simulink subsystem "Cell"  (R2019b)
settings: Solver=VariableStepAuto  StartTime=0.0  StopTime=10.0  RelTol=1e-3
libraries: nesl_utility x12, fl_lib x11, ee_lib x2
settings Model: Creator=PcElettronicaDynamis  LastModifiedBy=PcElettronicaDynamis

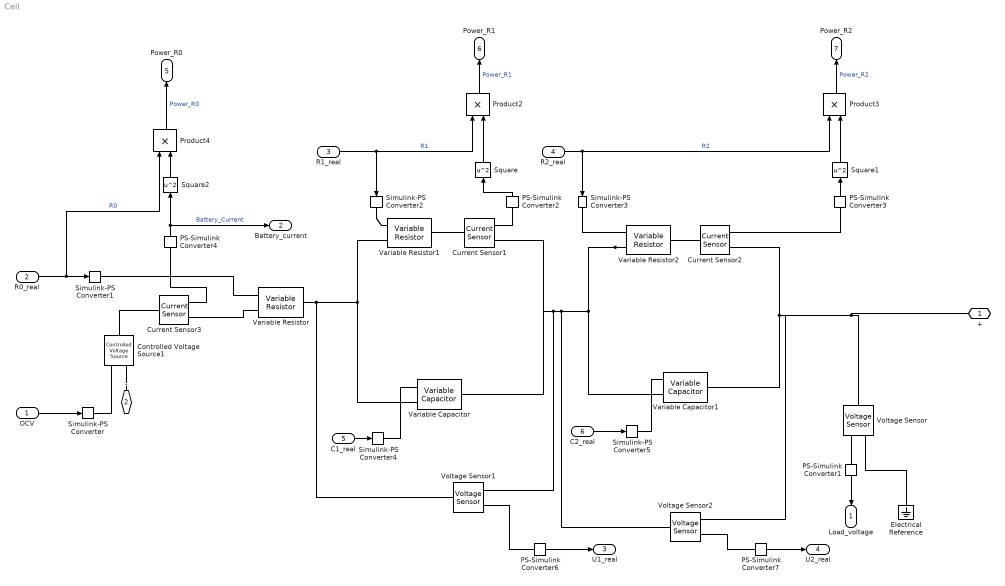
== system Cell ==
  OCV : Inport
  R0_real : Inport  Port=2
  R1_real : Inport  Port=3
  R2_real : Inport  Port=4
  C1_real : Inport  Port=5
  C2_real : Inport  Port=6
  Controlled Voltage Source1 : fl_lib/Electrical/Electrical Sources/Controlled Voltage Source
  Current Sensor1 : fl_lib/Electrical/Electrical Sensors/Current Sensor
  Current Sensor2 : fl_lib/Electrical/Electrical Sensors/Current Sensor
  Current Sensor3 : fl_lib/Electrical/Electrical Sensors/Current Sensor
  Electrical Reference : fl_lib/Electrical/Electrical Elements/Electrical Reference
  PS-Simulink Converter{1..4} (4 alike) : nesl_utility/PS-Simulink Converter  PhysicalDomain=network_engine_domain  SubClassName=ps_output  LeftPortType=input  RightPortType=output  PseudoPeriodic=off  Frequencies=[]  Unit=1  AffineConversion=off
  PS-Simulink Converter6 : nesl_utility/PS-Simulink Converter  PhysicalDomain=network_engine_domain  SubClassName=ps_output  LeftPortType=input  RightPortType=output  PseudoPeriodic=off  Frequencies=[]  Unit=inherit  AffineConversion=off
  PS-Simulink Converter7 : nesl_utility/PS-Simulink Converter  PhysicalDomain=network_engine_domain  SubClassName=ps_output  LeftPortType=input  RightPortType=output  PseudoPeriodic=off  Frequencies=[]  Unit=inherit  AffineConversion=off
  Product2 : Product
  Product3 : Product
  Product4 : Product
  Simulink-PS Converter{,1..5} (6 alike) : nesl_utility/Simulink-PS Converter  PhysicalDomain=network_engine_domain  SubClassName=ps_input  LeftPortType=input  RightPortType=output  PseudoPeriodic=off  Frequencies=[]  NoiseDistribution=none  NoiseParameters=[]  Unit=1  AffineConversion=off  FilteringAndDerivatives=provide  SimscapeFilterOrder=1  InputFilterTimeConstant=0.001  UdotUserProvided=0
  Square : Math  Operator=square  SaturateOnIntegerOverflow=on
  Square1 : Math  Operator=square  SaturateOnIntegerOverflow=on
  Square2 : Math  Operator=square  SaturateOnIntegerOverflow=on
  Variable Capacitor : ee_lib/Passive/Variable Capacitor  prm=2  Cmin=1e-9 F  r=1e-6 Ohm  v0=0 V  q0=0 C
      settings: SourceProductName=Simscape Electrical  SourceProductBaseCode=PS  InternalSimscapePortConfiguration="{\"Bottom\":[],\"Left\":[{\"id\":\"C\",\"label\":\"C\",\"type\":\"input\"},{\"id\":\"p\",\"label\":\"+\",\"type\":\"foundation.electrical.electrical\"}],\"Right\":[{\"id\":\"n\",\"label\":\"-\",\"type\":\"foundation.electrical.electrical\"}],\"Top\":[]}"
  Variable Capacitor1 : ee_lib/Passive/Variable Capacitor  prm=2  Cmin=1e-9 F  r=1e-6 Ohm  v0=0 V  q0=0 C
      settings: SourceProductName=Simscape Electrical  SourceProductBaseCode=PS  InternalSimscapePortConfiguration="{\"Bottom\":[],\"Left\":[{\"id\":\"C\",\"label\":\"C\",\"type\":\"input\"},{\"id\":\"p\",\"label\":\"+\",\"type\":\"foundation.electrical.electrical\"}],\"Right\":[{\"id\":\"n\",\"label\":\"-\",\"type\":\"foundation.electrical.electrical\"}],\"Top\":[]}"
  Variable Resistor : fl_lib/Electrical/Electrical Elements/Variable Resistor  Rmin=0 Ohm  i_specify=off  i_priority=None  i=0 A  i_nominal_specify=off  i_nominal_unit=A  i_nominal_value=1  v_specify=off  v_priority=None  v=0 V  v_nominal_specify=off  v_nominal_unit=V  v_nominal_value=1
  Variable Resistor1 : fl_lib/Electrical/Electrical Elements/Variable Resistor  Rmin=0 Ohm  i_specify=off  i_priority=None  i=0 A  i_nominal_specify=off  i_nominal_unit=A  i_nominal_value=1  v_specify=off  v_priority=None  v=0 V  v_nominal_specify=off  v_nominal_unit=V  v_nominal_value=1
  Variable Resistor2 : fl_lib/Electrical/Electrical Elements/Variable Resistor  Rmin=0 Ohm  i_specify=off  i_priority=None  i=0 A  i_nominal_specify=off  i_nominal_unit=A  i_nominal_value=1  v_specify=off  v_priority=None  v=0 V  v_nominal_specify=off  v_nominal_unit=V  v_nominal_value=1
  Voltage Sensor : fl_lib/Electrical/Electrical Sensors/Voltage Sensor
  Voltage Sensor1 : fl_lib/Electrical/Electrical Sensors/Voltage Sensor
  Voltage Sensor2 : fl_lib/Electrical/Electrical Sensors/Voltage Sensor
  + : PMIOPort  Side=Right
  - : PMIOPort  Port=2  Side=Right
  Load_voltage : Outport  VectorParamsAs1DForOutWhenUnconnected=off
  Battery_current : Outport  Port=2  VectorParamsAs1DForOutWhenUnconnected=off
  U1_real : Outport  Port=3
  U2_real : Outport  Port=4
  "Power_R0 " : Outport  Port=5  SignalName=Power_R0
  Power_R1 : Outport  Port=6  SignalName=Power_R0
  Power_R2 : Outport  Port=7  SignalName=Power_R2
  wires:
  Square/1 -> Product2/2
  C1_real/1 -> Simulink-PS Converter4/1
  Square1/1 -> Product3/2
  PS-Simulink Converter3/1 -> Square1/1
  PS-Simulink Converter2/1 -> Square/1
  PS-Simulink Converter1/1 -> Load_voltage/1
  OCV/1 -> Simulink-PS Converter/1
  PS-Simulink Converter6/1 -> U1_real/1
  Product2/1 -> Power_R1/1  "Power_R1"
  C2_real/1 -> Simulink-PS Converter5/1
  Product3/1 -> Power_R2/1  "Power_R2"
  R2_real/1 -> Product3/1, Simulink-PS Converter3/1  "R2"
  R1_real/1 -> Simulink-PS Converter2/1, Product2/1  "R1"
  Square2/1 -> Product4/2
  Product4/1 -> "Power_R0 "/1  "Power_R0"
  R0_real/1 -> Simulink-PS Converter1/1, Product4/1  "R0"
  PS-Simulink Converter7/1 -> U2_real/1
  PS-Simulink Converter4/1 -> Battery_current/1, Square2/1  "Battery_Current"
  connections:
  Variable Resistor2/LConn2 -- Variable Capacitor/RConn1 -- Current Sensor1/RConn2 -- Voltage Sensor1/RConn2 -- Voltage Sensor2/LConn1 -- Variable Capacitor1/LConn2
  Voltage Sensor1/LConn1 -- Variable Resistor1/LConn2 -- Variable Capacitor/LConn2 -- Variable Resistor/RConn1
  Current Sensor2/RConn2 -- +/RConn1 -- Voltage Sensor/LConn1 -- Voltage Sensor2/RConn2 -- Variable Capacitor1/RConn1
  Controlled Voltage Source1/LConn1 -- Current Sensor3/LConn1
  Simulink-PS Converter/RConn1 -- Controlled Voltage Source1/RConn1
  Voltage Sensor/RConn1 -- PS-Simulink Converter1/LConn1
  Voltage Sensor1/RConn1 -- PS-Simulink Converter6/LConn1
  Simulink-PS Converter4/RConn1 -- Variable Capacitor/LConn1
  Simulink-PS Converter3/RConn1 -- Variable Resistor2/LConn1
  Variable Resistor1/RConn1 -- Current Sensor1/LConn1
  -/RConn1 -- Controlled Voltage Source1/RConn2
  Current Sensor2/LConn1 -- Variable Resistor2/RConn1
  Current Sensor3/RConn2 -- Variable Resistor/LConn2
  Current Sensor3/RConn1 -- PS-Simulink Converter4/LConn1
  Current Sensor2/RConn1 -- PS-Simulink Converter3/LConn1
  Electrical Reference/LConn1 -- Voltage Sensor/RConn2
  PS-Simulink Converter7/LConn1 -- Voltage Sensor2/RConn1
  Simulink-PS Converter5/RConn1 -- Variable Capacitor1/LConn1
  Current Sensor1/RConn1 -- PS-Simulink Converter2/LConn1
  Simulink-PS Converter1/RConn1 -- Variable Resistor/LConn1
  Simulink-PS Converter2/RConn1 -- Variable Resistor1/LConn1
